simulink model "sol6_cubic"  (R2021b)
settings: Solver=VariableStepAuto  StartTime=0.0  StopTime=1.5  RelTol=1e-3
PreLoadFcn:
  | initModelData
  | trajectoryData
  | controlPID
StartFcn:
  | controlPID
values from neighbouring files (symbols this model uses):
  B = Bm+(Kb*Km/R)    (= 0.0149065789474)    [MyData_for_1_and_2.m]    (also in MyData_for_3_4_and_5.m; MyData_for_5_and_6.m)
  Jm = 5.5e-4    (= 0.00055)    [MyData_for_1_and_2.m]    (also in MyData_for_3_4_and_5.m; MyData_for_5_and_6.m)
  Kd = (R/Km)*((2*Jm*w*zeta)-B)    (= 0.369819047619)    [MyData_for_1_and_2.m]    (also in MyData_for_3_4_and_5.m = 0.2902; MyData_for_5_and_6.m = 0.0513428571429)
  Km = 0.105    [MyData_for_1_and_2.m]    (also in MyData_for_3_4_and_5.m; MyData_for_5_and_6.m)
  Kp = (R/Km)*(Jm*(w^2))    (= 14.3314285714)    [MyData_for_1_and_2.m]    (also in MyData_for_3_4_and_5.m = 9.95238095238; MyData_for_5_and_6.m = 1.59238095238)
  R = 0.76    [MyData_for_1_and_2.m]    (also in MyData_for_3_4_and_5.m; MyData_for_5_and_6.m)
  r = 156    [MyData_for_1_and_2.m]    (also in MyData_for_3_4_and_5.m; MyData_for_5_and_6.m)
undefined symbols (not defined in the file or in its folder): Ki
settings Model: Creator=esdan  LastModifiedBy=munir
settings SolverCC: AlgebraicLoopSolver=TrustRegion
settings DebuggingCC: SFMachineParentedDataDiag=warning

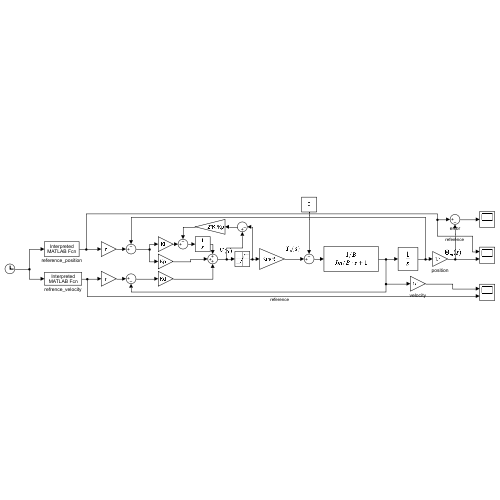
[thumbnail: Simulink's stored preview of the top-level diagram]
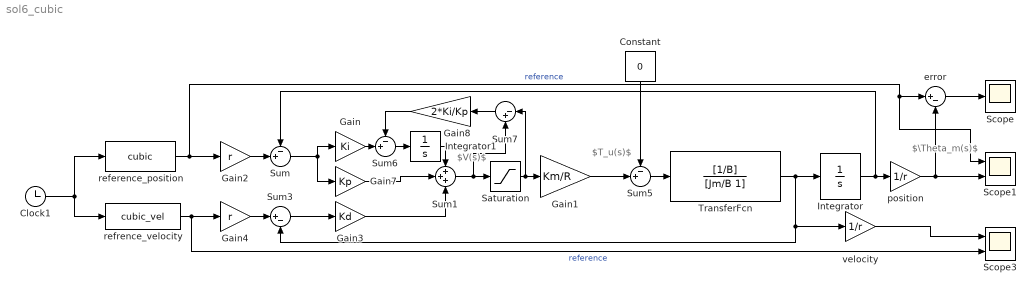
== system sol6_cubic ==
  note: $\Theta_m(s)$
  note: $V(s)$
  note: $T_u(s)$
  Clock1 : Clock
  Constant : Constant  Value=0
  Gain : Gain  Gain=Ki
  Gain1 : Gain  Gain=Km/R
  Gain2 : Gain  Gain=r
  Gain3 : Gain  Gain=Kd
  Gain4 : Gain  Gain=r
  Gain7 : Gain  Gain=Kp
  Gain8 : Gain  Gain=2*Ki/Kp
  Integrator : Integrator
  Integrator1 : Integrator
  Saturation : Saturate  UpperLimit=35  LowerLimit=-35
  Scope : Scope
  Scope1 : Scope  NumInputPorts=2
  Scope3 : Scope  NumInputPorts=2
  Sum : Sum  Inputs=-+|
  Sum1 : Sum  Inputs=+++
  Sum3 : Sum  Inputs=|+-
  Sum5 : Sum  Inputs=-+|
  Sum6 : Sum  Inputs=-+|
  Sum7 : Sum  Inputs=|-+
  TransferFcn : TransferFcn  Numerator=[1/B]  Denominator=[Jm/B 1]
  error : Sum  Inputs=|+-
  position : Gain  Gain=1/r
  reference_position : MATLABFcn  MATLABFcn=cubic
  refrence_velocity : MATLABFcn  MATLABFcn=cubic_vel
  velocity : Gain  Gain=1/r
  wires:
  TransferFcn/1 -> Integrator/1, velocity/1, Sum3/2
  Sum/1 -> Gain/1, Gain7/1
  Sum1/1 -> Sum7/2, Saturation/1
  Gain2/1 -> Sum/2
  reference_position/1 -> Gain2/1, error/1, Scope1/1  "reference"
  error/1 -> Scope/1
  Sum3/1 -> Gain3/1
  position/1 -> Scope1/2, error/2
  Integrator/1 -> Sum/1, position/1
  refrence_velocity/1 -> Gain4/1, Scope3/2  "reference"
  Gain4/1 -> Sum3/1
  velocity/1 -> Scope3/1
  Sum5/1 -> TransferFcn/1
  Gain1/1 -> Sum5/2
  Constant/1 -> Sum5/1
  Gain3/1 -> Sum1/3
  Gain7/1 -> Sum1/2
  Integrator1/1 -> Sum1/1
  Clock1/1 -> refrence_velocity/1, reference_position/1
  Gain8/1 -> Sum6/1
  Saturation/1 -> Sum7/1, Gain1/1
  Sum7/1 -> Gain8/1
  Gain/1 -> Sum6/2
  Sum6/1 -> Integrator1/1
